simulink model "HDLModulatorFull"  (R2024a)
settings: Solver=FixedStepDiscrete  StartTime=0.0  StopTime=stopTime  RelTol=1e-3
values from neighbouring files (symbols this model uses):
  dataSymbols = [ ... (first row only)    [testModulatorFull.m]
undefined symbols (not defined in the file or in its folder): fPHY, fs, numDataCarriers
libraries: hdlsllib x4, dspsrcs4 x4, HDL_ieee_8021513 x2, whdlutilities x1
settings Model: DataTypeOverride=Off  SimulationMode=accelerator  Creator=cotti  LastModifiedBy=cotti
settings OptimizationCC: BlockReduction=off  ConditionallyExecuteInputs=off  DefaultParameterBehavior=Inlined  InheritOutputTypeSmallerThanSingle=on
settings DebuggingCC: AlgebraicLoopMsg=error  ArtificialAlgebraicLoopMsg=error  SingleTaskRateTransMsg=error  UnconnectedInputMsg=warning  UnconnectedOutputMsg=warning  UnconnectedLineMsg=warning
settings HardwareCC: ProdBitPerPointer=32  ProdBitPerSizeT=32  ProdBitPerPtrDiffT=32  ProdLargestAtomicFloat=None  ProdIntDivRoundTo=Undefined  ProdEndianess=Unspecified  ProdWordSize=32  ProdHWDeviceType=ASIC/FPGA->ASIC/FPGA  TargetBitPerLong=64  TargetBitPerPointer=64  TargetBitPerSizeT=64  TargetBitPerPtrDiffT=64  TargetLongLongMode=on  TargetIntDivRoundTo=Zero  TargetEndianess=LittleEndian  TargetWordSize=64  TargetHWDeviceType=Custom Processor->MATLAB Host Computer  ProdEqTarget=off

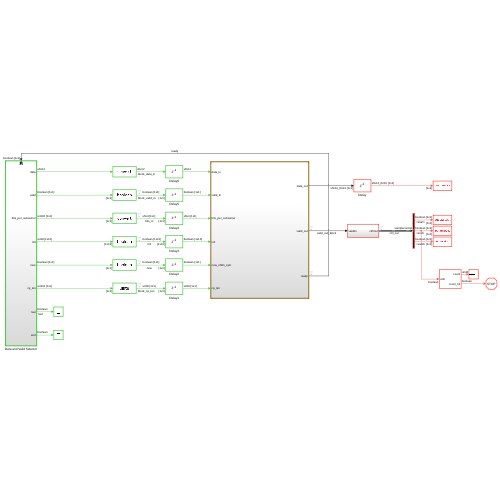
[thumbnail: Simulink's stored preview of the top-level diagram]
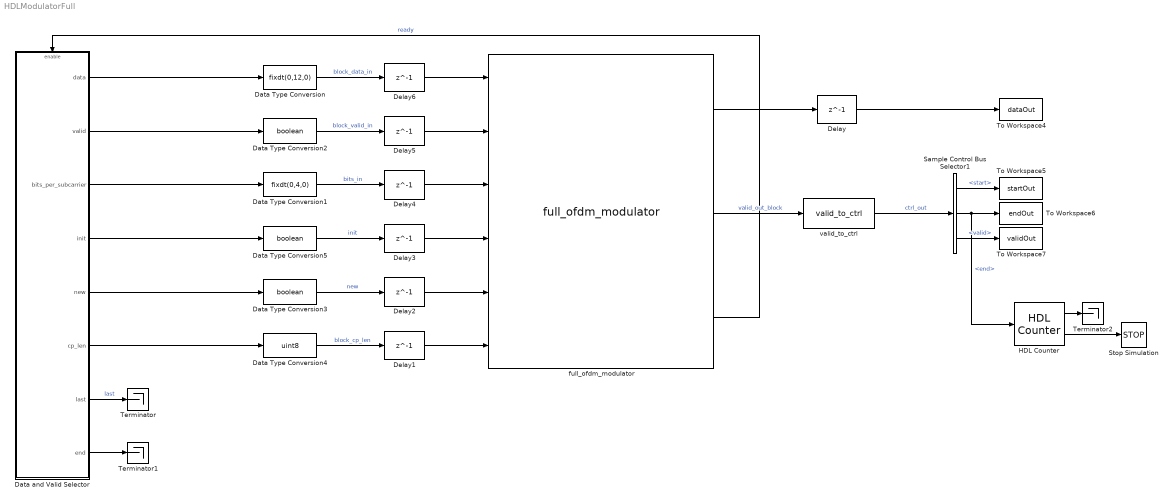
== system HDLModulatorFull ==
  Data Type Conversion : DataTypeConversion  OutDataTypeStr=fixdt(0,12,0)  SaturateOnIntegerOverflow=off  RndMeth=Floor  LockScale=on
  Data Type Conversion1 : DataTypeConversion  OutDataTypeStr=fixdt(0,4,0)  SaturateOnIntegerOverflow=off  RndMeth=Floor  LockScale=on
  Data Type Conversion2 : DataTypeConversion  OutDataTypeStr=boolean  SaturateOnIntegerOverflow=off  RndMeth=Floor  LockScale=on
  Data Type Conversion3 : DataTypeConversion  OutDataTypeStr=boolean  SaturateOnIntegerOverflow=off  RndMeth=Floor  LockScale=on
  Data Type Conversion4 : DataTypeConversion  OutDataTypeStr=uint8  SaturateOnIntegerOverflow=off  RndMeth=Floor  LockScale=on
  Data Type Conversion5 : DataTypeConversion  OutDataTypeStr=boolean  SaturateOnIntegerOverflow=off  RndMeth=Floor  LockScale=on
  Data and Valid Selector : Subsystem  TreatAsAtomicUnit=on
  Delay{,1..6} (7 alike) : Delay  DelayLength=1  InitialCondition=0  UseCircularBuffer=on
  HDL Counter : hdlsllib/Sources/HDL Counter  CountType=Count limited  CountInit=0  CountStep=1  CountMax=numberOfRepetitions  CountFromType=Initial value  CountFrom=0  CountResetPort=off  CountLoadPort=off  CountEnbPort=on  CountDirPort=off  CountHitOutputPort=on  CountDataType=Unsigned  CountWordLen=8  CountFracLen=0  CountSampTime=1
  Sample Control Bus Selector1 : whdlutilities/Sample Control Bus Selector  OutputSignals=start,end,valid
  Stop Simulation : Stop
  Terminator : Terminator
  Terminator1 : Terminator
  Terminator2 : Terminator
  To Workspace4 : ToWorkspace  VariableName=dataOut  SampleTime=1/fs
      settings: Save2DSignal=2-D array (concatenate along first dimension)
  To Workspace5 : ToWorkspace  VariableName=startOut  SampleTime=1/fs
      settings: Save2DSignal=2-D array (concatenate along first dimension)
  To Workspace6 : ToWorkspace  VariableName=endOut  SampleTime=1/fs
      settings: Save2DSignal=2-D array (concatenate along first dimension)
  To Workspace7 : ToWorkspace  VariableName=validOut  SampleTime=1/fs
      settings: Save2DSignal=2-D array (concatenate along first dimension)
  full_ofdm_modulator : HDL_ieee_8021513/full_ofdm_modulator  SystemSampleTime=-1  VariantActivationTime=update diagram  AllowFlexibleInterface=on  Latency=0  AutoFrameSizeCalculation=off
      settings: SourceProductName=HDL IEEE 8021513
  valid_to_ctrl : HDL_ieee_8021513/valid_to_ctrl  SystemSampleTime=-1  VariantActivationTime=update diagram  AllowFlexibleInterface=on  Latency=0  AutoFrameSizeCalculation=off
      settings: SourceProductName=HDL IEEE 8021513
  wires:
  full_ofdm_modulator/2 -> valid_to_ctrl/1  "valid_out_block"
  full_ofdm_modulator/1 -> Delay/1
  Sample Control Bus Selector1/3 -> To Workspace7/1  "<valid>"
  valid_to_ctrl/1 -> Sample Control Bus Selector1/1  "ctrl_out"
  Sample Control Bus Selector1/1 -> To Workspace5/1  "<start>"
  Sample Control Bus Selector1/2 -> HDL Counter/1, To Workspace6/1  "<end>"
  Data Type Conversion1/1 -> Delay4/1  "bits_in"
  Data and Valid Selector/8(end) -> Terminator1/1
  Data Type Conversion2/1 -> Delay5/1  "block_valid_in"
  Data Type Conversion4/1 -> Delay1/1  "block_cp_len"
  Data and Valid Selector/6(cp_len) -> Data Type Conversion4/1
  Data and Valid Selector/4(init) -> Data Type Conversion5/1
  Data and Valid Selector/2(valid) -> Data Type Conversion2/1
  Data Type Conversion/1 -> Delay6/1  "block_data_in"
  Data and Valid Selector/1(data) -> Data Type Conversion/1
  Data and Valid Selector/3(bits_per_subcarrier) -> Data Type Conversion1/1
  Data and Valid Selector/5(new) -> Data Type Conversion3/1
  Data and Valid Selector/7(last) -> Terminator/1  "last"
  Data Type Conversion3/1 -> Delay2/1  "new"
  Data Type Conversion5/1 -> Delay3/1  "init"
  full_ofdm_modulator/3 -> Data and Valid Selector/Enable  "ready"
  Delay/1 -> To Workspace4/1
  HDL Counter/1 -> Terminator2/1
  HDL Counter/2 -> Stop Simulation/1
  Delay1/1 -> full_ofdm_modulator/6
  Delay2/1 -> full_ofdm_modulator/5
  Delay3/1 -> full_ofdm_modulator/4
  Delay4/1 -> full_ofdm_modulator/3
  Delay5/1 -> full_ofdm_modulator/2
  Delay6/1 -> full_ofdm_modulator/1

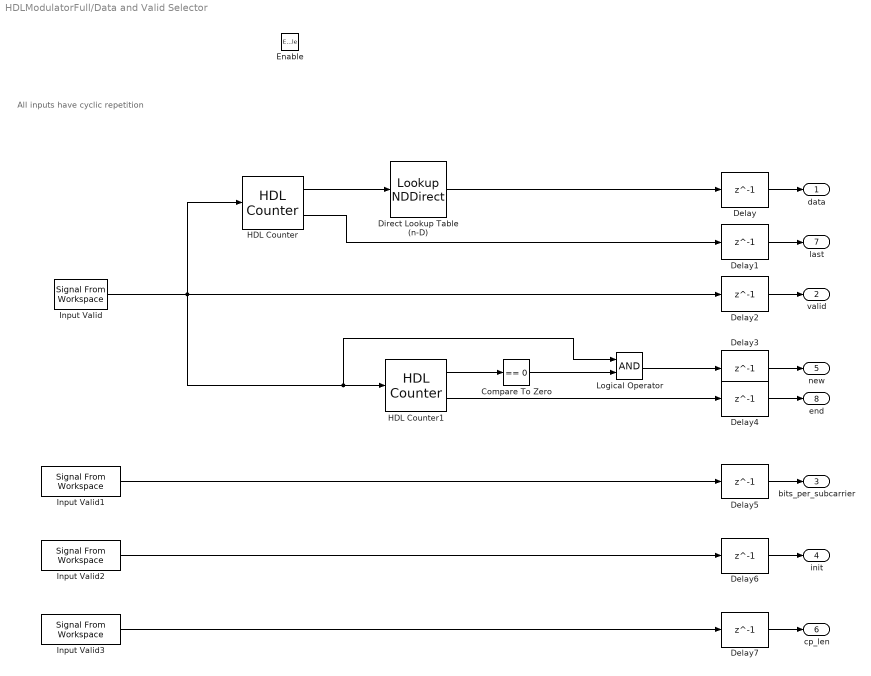
== system HDLModulatorFull/Data and Valid Selector ==
  note: All inputs have cyclic repetition
  Enable : EnablePort
  Compare To Zero : hdlsllib/Logic and Bit Operations/Compare To Zero  relop===  OutDataTypeStr=boolean
  Delay{,1..7} (8 alike) : Delay  DelayLength=1  InitialCondition=0  UseCircularBuffer=on
  Direct Lookup Table (n-D) : LookupNDDirect  NumberOfTableDimensions=1  Table=dataSymbols  DiagnosticForOutOfRangeInput=Error  TableDataTypeStr=fixdt(0,12,0)
  HDL Counter : hdlsllib/Sources/HDL Counter  CountType=Count limited  CountInit=0  CountStep=1  CountMax=length(dataSymbols) -1  CountFromType=Initial value  CountFrom=0  CountResetPort=off  CountLoadPort=off  CountEnbPort=on  CountDirPort=off  CountHitOutputPort=on  CountDataType=Unsigned  CountWordLen=nextpow2(length(dataSymbols))  CountFracLen=0  CountSampTime=1
  HDL Counter1 : hdlsllib/Sources/HDL Counter  CountType=Count limited  CountInit=0  CountStep=1  CountMax=numDataCarriers-1  CountFromType=Initial value  CountFrom=0  CountResetPort=off  CountLoadPort=off  CountEnbPort=on  CountDirPort=off  CountHitOutputPort=on  CountDataType=Unsigned  CountWordLen=nextpow2(numDataCarriers)  CountFracLen=0  CountSampTime=1
  Input Valid : dspsrcs4/Signal From Workspace  X=validIn  Ts=1/fPHY  nsamps=1  OutputAfterFinalValue=Cyclic repetition  ignoreOrWarnInputAndFrameLengths=off  OutputFrames=off
  Input Valid1 : dspsrcs4/Signal From Workspace  X=bitsPerSubcarrier  Ts=1/fPHY  nsamps=1  OutputAfterFinalValue=Cyclic repetition  ignoreOrWarnInputAndFrameLengths=off  OutputFrames=off
  Input Valid2 : dspsrcs4/Signal From Workspace  X=init  Ts=1/fPHY  nsamps=1  OutputAfterFinalValue=Cyclic repetition  ignoreOrWarnInputAndFrameLengths=off  OutputFrames=off
  Input Valid3 : dspsrcs4/Signal From Workspace  X=cpLen  Ts=1/fPHY  nsamps=1  OutputAfterFinalValue=Cyclic repetition  ignoreOrWarnInputAndFrameLengths=off  OutputFrames=off
  Logical Operator : Logic  AllPortsSameDT=off  OutDataTypeStr=boolean
  data : Outport  InitialOutput=0  VectorParamsAs1DForOutWhenUnconnected=off
  valid : Outport  Port=2  InitialOutput=0  VectorParamsAs1DForOutWhenUnconnected=off
  bits_per_subcarrier : Outport  Port=3  VectorParamsAs1DForOutWhenUnconnected=off
  init : Outport  Port=4  VectorParamsAs1DForOutWhenUnconnected=off
  new : Outport  Port=5  VectorParamsAs1DForOutWhenUnconnected=off
  cp_len : Outport  Port=6  VectorParamsAs1DForOutWhenUnconnected=off
  last : Outport  Port=7  VectorParamsAs1DForOutWhenUnconnected=off
  end : Outport  Port=8  VectorParamsAs1DForOutWhenUnconnected=off
  wires:
  HDL Counter/1 -> Direct Lookup Table (n-D)/1
  Direct Lookup Table (n-D)/1 -> Delay/1
  HDL Counter/2 -> Delay1/1
  HDL Counter1/1 -> Compare To Zero/1
  Compare To Zero/1 -> Logical Operator/2
  Logical Operator/1 -> Delay3/1
  HDL Counter1/2 -> Delay4/1
  Input Valid/1 -> HDL Counter/1, Delay2/1, Logical Operator/1, HDL Counter1/1
  Input Valid3/1 -> Delay7/1
  Input Valid2/1 -> Delay6/1
  Input Valid1/1 -> Delay5/1
  Delay/1 -> data/1
  Delay1/1 -> last/1
  Delay2/1 -> valid/1
  Delay3/1 -> new/1
  Delay4/1 -> end/1
  Delay5/1 -> bits_per_subcarrier/1
  Delay6/1 -> init/1
  Delay7/1 -> cp_len/1
